simulink model "cruise_h8000_u250"  (R2023b)
settings: Solver=ode3  StartTime=0.0  StopTime=300  FixedStep=0.01  RelTol=1e-3
undefined symbols (not defined in the file or in its folder): cruise_h8000_u250
settings Model: Creator=Pro14  LastModifiedBy=阿汪
settings SolverCC: AlgebraicLoopSolver=TrustRegion
settings RTWCC: GPUComputeCapability=5.0  DLArmComputeVersion=19.05

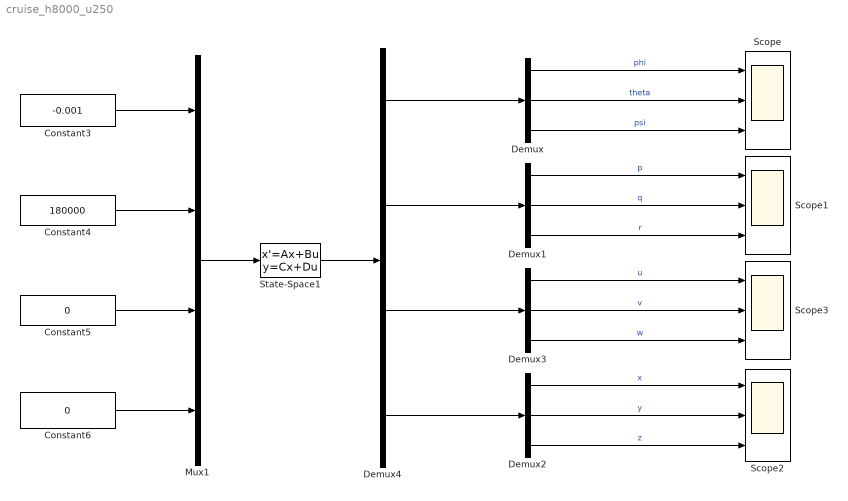
== system cruise_h8000_u250 ==
  Constant3 : Constant  Value=-0.001
  Constant4 : Constant  Value=180000
  Constant5 : Constant  Value=0
  Constant6 : Constant  Value=0
  Demux{,1..3} (4 alike) : Demux  Outputs=3
  Demux4 : Demux
  Mux1 : Mux
  Scope{,1..3} (4 alike) : Scope  NumInputPorts=3
  State-Space1 : StateSpace  A=cruise_h8000_u250.A  B=cruise_h8000_u250.B  C=cruise_h8000_u250.C  D=cruise_h8000_u250.D  InitialCondition=[0;0.001;0;0;0;0;250;0;0.1;0;0;-8000]
  wires:
  State-Space1/1 -> Demux4/1
  Demux3/3 -> Scope3/3  "w"
  Demux2/1 -> Scope2/1  "x"
  Demux4/2 -> Demux1/1
  Demux3/2 -> Scope3/2  "v"
  Constant3/1 -> Mux1/1
  Constant4/1 -> Mux1/2
  Demux3/1 -> Scope3/1  "u"
  Demux1/2 -> Scope1/2  "q"
  Demux1/3 -> Scope1/3  "r"
  Constant6/1 -> Mux1/4
  Demux4/3 -> Demux3/1
  Demux/1 -> Scope/1  "phi"
  Demux4/4 -> Demux2/1
  Demux1/1 -> Scope1/1  "p"
  Demux4/1 -> Demux/1
  Demux/2 -> Scope/2  "theta"
  Demux/3 -> Scope/3  "psi"
  Mux1/1 -> State-Space1/1
  Demux2/3 -> Scope2/3  "z"
  Constant5/1 -> Mux1/3
  Demux2/2 -> Scope2/2  "y"
